simulink model "simple_force_nullspace_control"  (R2021b)
settings: Solver=VariableStepAuto  StartTime=0.0  StopTime=10.0  RelTol=1e-3
values from neighbouring files (symbols this model uses):
  a = [-2.0 2.0 ... (first row only)    [init.m]
  A_p = [0 1 0 0 0 0 ... (first row only)    [init.m]
  b = [-0.05 0.1 ... (first row only)    [init.m]
  B_p = [0     0     0 ... (first row only)    [init.m]
  f_max = 200*ones(m,1)    [init.m]
  f_min = 10*ones(m,1)    [init.m]
  f_ref = 0.5*(f_min+f_max)    [init.m]
  l = inverseKinematics(a, b, x, m)    [init.m]
  m = 4    [init.m]
  x = [r; 0]    [init.m]
  x_ss_0 = [x(1); 0; x(2); 0; x(3);0]    [init.m]
undefined symbols (not defined in the file or in its folder): DiscIntNeverNeededParam
settings Model: Creator=Sølve  LastModifiedBy=Sølve

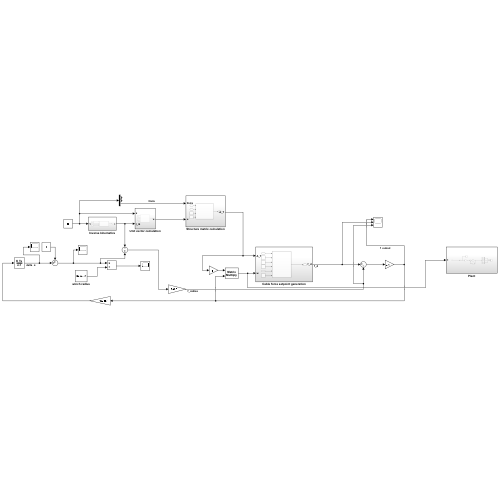
[thumbnail: Simulink's stored preview of the top-level diagram]
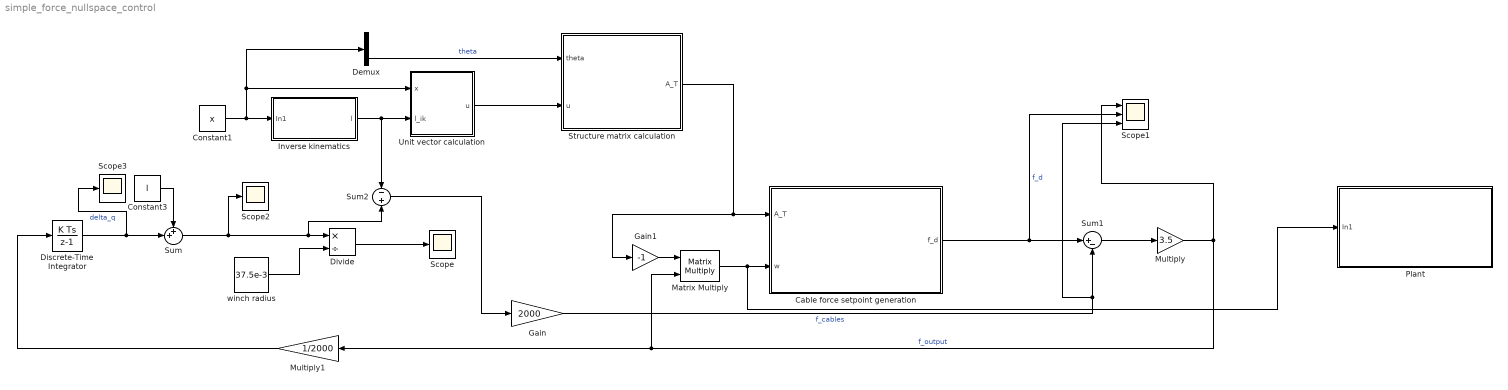
== system simple_force_nullspace_control ==
  Cable force setpoint generation : Subsystem
  Constant1 : Constant  Value=x
  Constant3 : Constant  Value=l
  Demux : Demux  Outputs=3
  Discrete-Time Integrator : DiscreteIntegrator  gainval=1  SampleTime=-1  ICPrevOutput=DiscIntNeverNeededParam  ICPrevScaledInput=DiscIntNeverNeededParam
  Divide : Product  Inputs=*/
  Gain : Gain  Gain=2000
  Gain1 : Gain  Gain=-1
  Inverse kinematics : Subsystem
  Matrix Multiply : Product  Multiplication=Matrix(*)
  Multiply : Gain  Gain=3.5
  Multiply1 : Gain  Gain=1/2000
  Plant : Subsystem
  Scope : Scope
  Scope1 : Scope  NumInputPorts=3
  Scope2 : Scope
  Scope3 : Scope
  Structure matrix calculation : Subsystem
  Sum : Sum  Inputs=++|
  Sum1 : Sum  Inputs=|+-
  Sum2 : Sum  Inputs=-|+
  Unit vector calculation : Subsystem
  winch radius : Constant  Value=37.5e-3
  wires:
  winch radius/1 -> Divide/2
  Divide/1 -> Scope/1
  Constant3/1 -> Sum/1
  Constant1/1 -> Demux/1, Unit vector calculation/1(x), Inverse kinematics/1(In1)
  Demux/3 -> Structure matrix calculation/1(theta)  "theta"
  Unit vector calculation/1(u) -> Structure matrix calculation/2(u)
  Inverse kinematics/1(l) -> Unit vector calculation/2(l_ik), Sum2/1
  Structure matrix calculation/1(A_T) -> Gain1/1, Cable force setpoint generation/1(A_T)
  Cable force setpoint generation/1(f_d) -> Scope1/2, Sum1/1  "f_d"
  Multiply/1 -> Scope1/1, Matrix Multiply/2, Multiply1/1  "f_output"
  Sum2/1 -> Gain/1
  Gain/1 -> Sum1/2, Scope1/3  "f_cables"
  Sum1/1 -> Multiply/1
  Multiply1/1 -> Discrete-Time Integrator/1
  Discrete-Time Integrator/1 -> Scope3/1, Sum/2  "delta_q"
  Sum/1 -> Scope2/1, Sum2/2, Divide/1
  Gain1/1 -> Matrix Multiply/1
  Matrix Multiply/1 -> Plant/1(In1), Cable force setpoint generation/2(w)

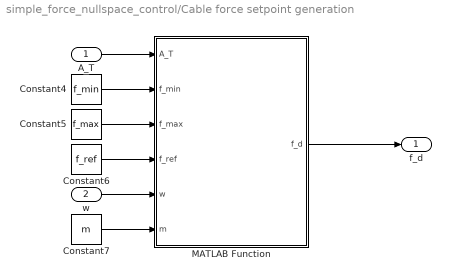
== system simple_force_nullspace_control/Cable force setpoint generation ==
  A_T : Inport
  w : Inport  Port=2
  Constant4 : Constant  Value=f_min
  Constant5 : Constant  Value=f_max
  Constant6 : Constant  Value=f_ref
  Constant7 : Constant  Value=m
  MATLAB Function : MATLAB Function  TreatAsAtomicUnit=on
  f_d : Outport
  wires:
  w/1 -> MATLAB Function/5(w)
  Constant5/1 -> MATLAB Function/3(f_max)
  Constant6/1 -> MATLAB Function/4(f_ref)
  Constant7/1 -> MATLAB Function/6(m)
  A_T/1 -> MATLAB Function/1(A_T)
  MATLAB Function/1(f_d) -> f_d/1
  Constant4/1 -> MATLAB Function/2(f_min)

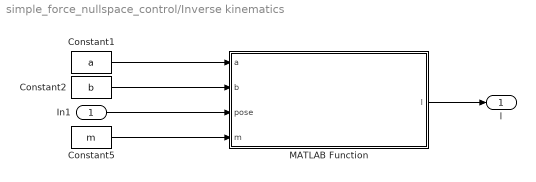
== system simple_force_nullspace_control/Inverse kinematics ==
  In1 : Inport
  Constant1 : Constant  Value=a
  Constant2 : Constant  Value=b
  Constant5 : Constant  Value=m
  MATLAB Function : MATLAB Function  TreatAsAtomicUnit=on
  l : Outport
  wires:
  MATLAB Function/1(l) -> l/1
  Constant2/1 -> MATLAB Function/2(b)
  In1/1 -> MATLAB Function/3(pose)
  Constant5/1 -> MATLAB Function/4(m)
  Constant1/1 -> MATLAB Function/1(a)

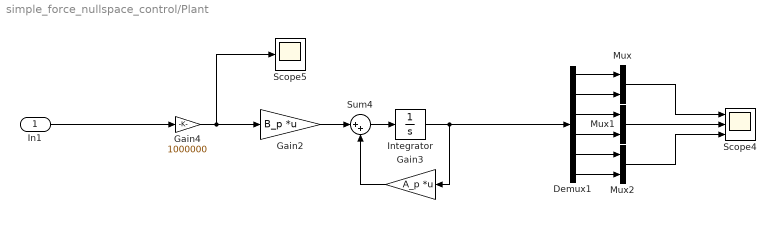
== system simple_force_nullspace_control/Plant ==
  In1 : Inport
  Demux1 : Demux  Outputs=6
  Gain2 : Gain  Gain=B_p  Multiplication=Matrix(K*u)
  Gain3 : Gain  Gain=A_p  Multiplication=Matrix(K*u)
  Gain4 : Gain  Gain=1000000
  Integrator : Integrator  InitialCondition=x_ss_0
  Mux : Mux  Inputs=2
  Mux1 : Mux  Inputs=2
  Mux2 : Mux  Inputs=2
  Scope4 : Scope  NumInputPorts=3
  Scope5 : Scope
  Sum4 : Sum  Inputs=|++
  wires:
  Integrator/1 -> Gain3/1, Demux1/1
  Demux1/4 -> Mux1/2
  Mux/1 -> Scope4/1
  Sum4/1 -> Integrator/1
  Demux1/2 -> Mux/2
  Gain2/1 -> Sum4/1
  Mux1/1 -> Scope4/2
  Gain4/1 -> Scope5/1, Gain2/1
  Demux1/1 -> Mux/1
  Gain3/1 -> Sum4/2
  Demux1/6 -> Mux2/2
  Demux1/5 -> Mux2/1
  Demux1/3 -> Mux1/1
  Mux2/1 -> Scope4/3
  In1/1 -> Gain4/1

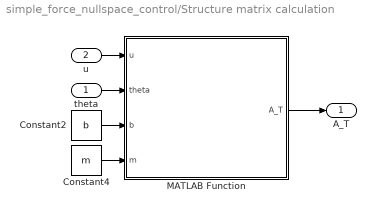
== system simple_force_nullspace_control/Structure matrix calculation ==
  theta : Inport
  u : Inport  Port=2
  Constant2 : Constant  Value=b
  Constant4 : Constant  Value=m
  MATLAB Function : MATLAB Function  TreatAsAtomicUnit=on
  A_T : Outport
  wires:
  Constant4/1 -> MATLAB Function/4(m)
  Constant2/1 -> MATLAB Function/3(b)
  theta/1 -> MATLAB Function/2(theta)
  MATLAB Function/1(A_T) -> A_T/1
  u/1 -> MATLAB Function/1(u)

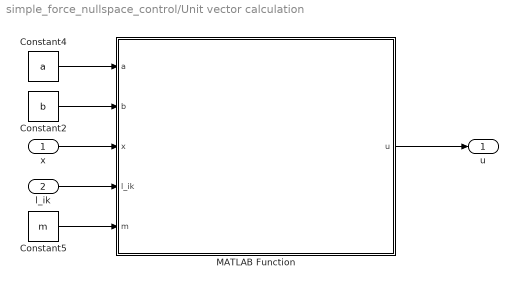
== system simple_force_nullspace_control/Unit vector calculation ==
  x : Inport
  l_ik : Inport  Port=2
  Constant2 : Constant  Value=b
  Constant4 : Constant  Value=a
  Constant5 : Constant  Value=m
  MATLAB Function : MATLAB Function  TreatAsAtomicUnit=on
  u : Outport
  wires:
  l_ik/1 -> MATLAB Function/4(l_ik)
  Constant2/1 -> MATLAB Function/2(b)
  x/1 -> MATLAB Function/3(x)
  Constant5/1 -> MATLAB Function/5(m)
  Constant4/1 -> MATLAB Function/1(a)
  MATLAB Function/1(u) -> u/1

== matlab function simple_force_nullspace_control/Unit vector calculation/MATLAB Function ==
  data: a input; u output; b input; x input; l_ik input; m input
function u = calculateCableUnitVectors(a, b, x, l_ik, m)
    l = a - x(1:2) - R_z(x(3))*b;
    u = zeros(2,4);
    for i=1:m
        u(:,i) = l(:,i)/l_ik(i);
    end
end

function R = R_z(theta)
    R = [cos(theta) -sin(theta);
         sin(theta)  cos(theta)];
end

== matlab function simple_force_nullspace_control/Inverse kinematics/MATLAB Function ==
  data: a input; l output; b input; pose input; m input
function l = inverseKinematics(a, b, pose, m)
    x     = pose(1);
    y     = pose(2);
    theta = pose(3);

    l = zeros(4,1);
    for i=1:m
        l(i) = norm(a(:,i)-[x;y]-R_z(theta)*b(:,i),2);
    end
end


function R = R_z(theta)
    R = [cos(theta) -sin(theta);
         sin(theta)  cos(theta)];
end

== matlab function simple_force_nullspace_control/Structure matrix calculation/MATLAB Function ==
  data: u input; A_T output; theta input; b input; m input
function A_T = calculateStructureMatrix(u, theta, b, m)
    crossProd = zeros(3, 4);
    for i=1:m
        crossProd(:,i) = cross([0;R_z(theta)*b(:,i);], [0;u(:,i)]);
    end
    A_T1 = [zeros(1,4);
           u;
           crossProd];
    A_T = A_T1(2:4,:);
end

function R = R_z(theta)
    R = [cos(theta) -sin(theta);
         sin(theta)  cos(theta)];
end

== matlab function simple_force_nullspace_control/Cable force setpoint generation/MATLAB Function ==
  data: A_T input; f_d output; f_min input; f_max input; f_ref input; w input; m input
function f_d = forceQP(A_T, f_min, f_max, f_ref, w, m)
    coder.extrinsic('quadprog');
    f_d = zeros(4,1);
    f_d = quadprog(eye(m),-f_ref,[],[],A_T, -w,f_min,f_max);
